simulink model "fsk_block_implementation_0"  (R2021a)
settings: Solver=VariableStepAuto  StartTime=0.0  StopTime=10  RelTol=1e-3
libraries: commchan3 x4, commsink2 x4, commdigbbndfm2 x4, commdigbbndpm3 x2, commdigbbndam3 x2, dspquant2 x2, commsrccod2 x1, dspsrcs4 x1, commrandsrc3 x1, dspsigops x1
settings Model: Creator=Yash  LastModifiedBy=Bharat Gunhalkar

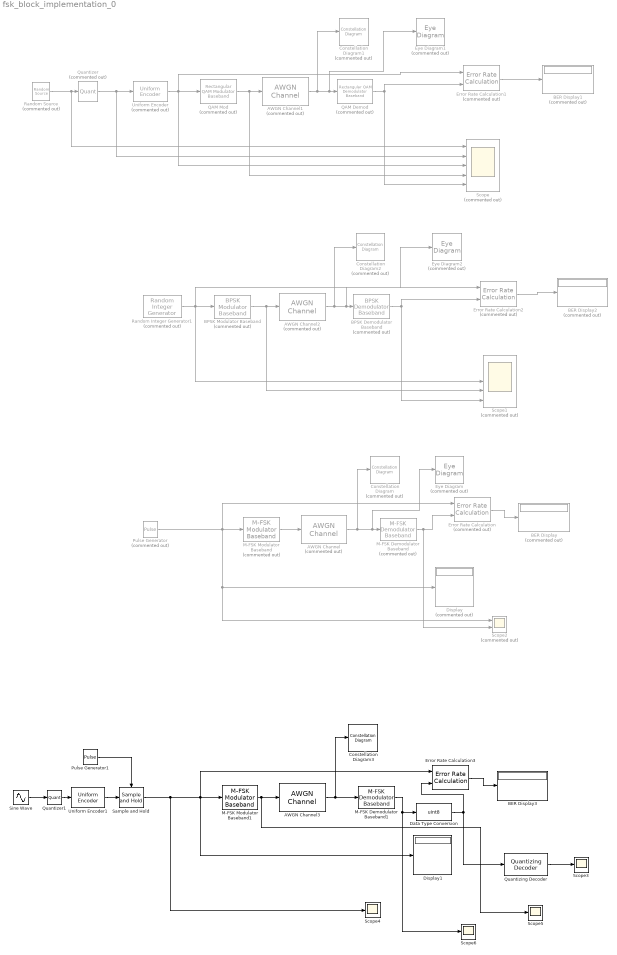
== system fsk_block_implementation_0 ==
  AWGN Channel : commchan3/AWGN Channel  Commented=on  InputProcessing=Columns as channels (frame based)  seed=67  noiseMode="Signal to noise ratio  (Eb/No)"  EbNodB=100  EsNodB=10  SNRdB=10  bitsPerSym=1  Ps=1  Tsym=1  variance=1
  AWGN Channel1 : commchan3/AWGN Channel  Commented=on  InputProcessing=Columns as channels (frame based)  seed=67  noiseMode="Signal to noise ratio  (Eb/No)"  EbNodB=-10  EsNodB=10  SNRdB=10  bitsPerSym=1  Ps=1  Tsym=1  variance=1
  AWGN Channel2 : commchan3/AWGN Channel  Commented=on  InputProcessing=Columns as channels (frame based)  seed=67  noiseMode="Signal to noise ratio  (Eb/No)"  EbNodB=-10  EsNodB=10  SNRdB=10  bitsPerSym=1  Ps=1  Tsym=1  variance=1
  AWGN Channel3 : commchan3/AWGN Channel  InputProcessing=Columns as channels (frame based)  seed=67  noiseMode="Signal to noise ratio  (Eb/No)"  EbNodB=100  EsNodB=10  SNRdB=10  bitsPerSym=1  Ps=1  Tsym=1  variance=1
  BER Display : Display  Commented=on
  BER Display1 : Display  Commented=on
  BER Display2 : Display  Commented=on
  BER Display3 : Display
  BPSK Demodulator Baseband : commdigbbndpm3/BPSK Demodulator Baseband  Commented=on  DecType=Hard decision  VarSource=Dialog  Variance=1  Ph=0  outDtype=Inherit via internal rule  derotateFactorWordLen=16  derotateFactorDataTypeStr=Inherit: Same word length as input  derotateFactorLastDataTypeStr=Inherit: Same word length as input
  BPSK Modulator Baseband : commdigbbndpm3/BPSK Modulator Baseband  Commented=on  Ph=0  outDtype=double  outWordLen=16  outUDDataType=sfix(16)  outFracLenMode=Best precision  outFracLen=15  outDataTypeStr=double  outLastDataTypeStr=double
  Constellation Diagram : ConstellationDiagram  Commented=on
  Constellation Diagram1 : ConstellationDiagram  Commented=on
  Constellation Diagram2 : ConstellationDiagram  Commented=on
  Constellation Diagram3 : ConstellationDiagram
  Data Type Conversion : DataTypeConversion  OutDataTypeStr=uint8
  Display : Display  Commented=on
  Display1 : Display
  Error Rate Calculation : commsink2/Error Rate Calculation  Commented=on  N=0  st_delay=0  cp_mode=Entire frame  subframe=[]  PMode=Port  WsName=ErrorVec  RsMode2=off  stop=off  numErr=100  maxBits=1e6
  Error Rate Calculation1 : commsink2/Error Rate Calculation  Commented=on  N=0  st_delay=0  cp_mode=Entire frame  subframe=[]  PMode=Port  WsName=ErrorVec  RsMode2=off  stop=off  numErr=100  maxBits=1e6
  Error Rate Calculation2 : commsink2/Error Rate Calculation  Commented=on  N=0  st_delay=0  cp_mode=Entire frame  subframe=[]  PMode=Port  WsName=ErrorVec  RsMode2=off  stop=off  numErr=100  maxBits=1e6
  Error Rate Calculation3 : commsink2/Error Rate Calculation  N=0  st_delay=0  cp_mode=Entire frame  subframe=[]  PMode=Port  WsName=ErrorVec  RsMode2=off  stop=off  numErr=100  maxBits=1e6
  Eye Diagram : EyeDiagram  Commented=on
  Eye Diagram1 : EyeDiagram  Commented=on
  Eye Diagram2 : EyeDiagram  Commented=on
  M-FSK Demodulator Baseband : commdigbbndfm2/M-FSK Demodulator Baseband  Commented=on  M=8  OutType=Integer  Dec=Gray  freqSep=6  numSamp=17  RateOptions=Enforce single-rate processing  outDataType=double
      settings: SourceProductBaseCode=CM
  M-FSK Demodulator Baseband1 : commdigbbndfm2/M-FSK Demodulator Baseband  M=8  OutType=Integer  Dec=Gray  freqSep=6  numSamp=17  RateOptions=Enforce single-rate processing  outDataType=double
      settings: SourceProductBaseCode=CM
  M-FSK Modulator Baseband : commdigbbndfm2/M-FSK Modulator Baseband  Commented=on  M=8  InType=Integer  Enc=Gray  freqSep=6  phaseType=Continuous  numSamp=17  RateOptions=Enforce single-rate processing  outDataType=double
  M-FSK Modulator Baseband1 : commdigbbndfm2/M-FSK Modulator Baseband  M=8  InType=Integer  Enc=Gray  freqSep=6  phaseType=Continuous  numSamp=17  RateOptions=Enforce single-rate processing  outDataType=double
  Pulse Generator : DiscretePulseGenerator  Commented=on  Amplitude=5  SampleTime=0.0001
  Pulse Generator1 : DiscretePulseGenerator  SampleTime=0.001
  QAM Demod : commdigbbndam3/Rectangular QAM Demodulator Baseband  Commented=on  M=16  OutType=Integer  DecType=Hard decision  VarSource=Dialog  Variance=1  Dec=Gray  Mapping=[0:15]  PowType=Min. distance between symbols  MinDist=2  AvgPow=1  PeakPow=1  Ph=0  outDtype1=Inherit via internal rule  outDtype2=Inherit via internal rule  derotateFactorWordLen=16  derotateFactorDataTypeStr=Inherit: Same word length as input  derotateFactorLastDataTypeStr=Inherit: Same word length as input  denormFactorWordLen=16  denormFactorDataTypeStr=Inherit: Same word length as input  denormFactorLastDataTypeStr=Inherit: Same word length as input  prodOutWordLen=32  prodOutOverflowMode=Wrap  prodOutRoundingMode=Floor  prodOutOvFlMode=off  prodOutOvFlModeLastStrValue=off  sumWordLen=32
  QAM Mod : commdigbbndam3/Rectangular QAM Modulator Baseband  Commented=on  M=16  InType=Integer  Enc=Gray  Mapping=[0:15]  PowType=Min. distance between symbols  MinDist=2  AvgPow=1  PeakPow=1  Ph=0  outDtype=double  outWordLen=16  outUDDataType=sfix(16)  outFracLenMode=Best precision  outFracLen=15  outDataTypeStr=double  outLastDataTypeStr=double
  Quantizer : Quantizer  Commented=on  QuantizationInterval=0.25  LinearizeAsGain=off
  Quantizer1 : Quantizer  QuantizationInterval=.333
  Quantizing Decoder : commsrccod2/Quantizing Decoder  codebook=[-.825 -.5 0, .5 .825]  QuDType=double
      settings: SourceProductBaseCode=CM
  Random Source : dspsrcs4/Random Source  Commented=on  SrcType=Uniform  NormMethod=Ziggurat  CltLength=12  MinVal=0  MaxVal=1  MeanVal=0  VarVal=1  RepMode=Not repeatable  rawSeed=1  IsInherit=off  SampMode=Discrete  SampTime=0.1  SampFrame=1  DataType=Single  OutComplex=Real  OutputFrames=off
  Random Integer Generator1 : commrandsrc3/Random Integer Generator  Commented=on  SetSize=2  SeedSource=Auto  Seed=0  SampleTime=0.1  SamplesPerFrame=1  OutputDataType=double  SimulateUsing=Interpreted execution
  Sample and Hold : dspsigops/Sample and Hold  trig=Rising edge  initCond=0  latchinput=off
  Scope : Scope  Commented=on  NumInputPorts=5
  Scope1 : Scope  Commented=on  NumInputPorts=5
  Scope2 : Scope  Commented=on  NumInputPorts=2
  Scope{3..6} (4 alike) : Scope
  Sine Wave : Sin  Amplitude=5  Frequency=2*pi  SampleTime=0.001
  Uniform Encoder : dspquant2/Uniform Encoder  Commented=on  peak=1  bits=4  otype=Unsigned integer
  Uniform Encoder1 : dspquant2/Uniform Encoder  peak=1  bits=3  otype=Unsigned integer
  wires:
  Error Rate Calculation1/1 -> BER Display1/1
  QAM Mod/1 -> AWGN Channel1/1, Scope/4
  Quantizer/1 -> Uniform Encoder/1, Scope/2
  AWGN Channel1/1 -> Eye Diagram1/1, QAM Demod/1, Constellation Diagram1/1
  Uniform Encoder/1 -> QAM Mod/1, Error Rate Calculation1/1, Scope/3
  Random Source/1 -> Scope/1, Quantizer/1
  QAM Demod/1 -> Error Rate Calculation1/2, Scope/5
  Random Integer Generator1/1 -> BPSK Modulator Baseband/1, Error Rate Calculation2/1, Scope1/3
  AWGN Channel2/1 -> BPSK Demodulator Baseband/1, Eye Diagram2/1, Constellation Diagram2/1
  Error Rate Calculation2/1 -> BER Display2/1
  BPSK Demodulator Baseband/1 -> Error Rate Calculation2/2, Scope1/5
  BPSK Modulator Baseband/1 -> AWGN Channel2/1, Scope1/4
  AWGN Channel/1 -> Eye Diagram/1, M-FSK Demodulator Baseband/1, Constellation Diagram/1
  M-FSK Demodulator Baseband/1 -> Scope2/2, Error Rate Calculation/2
  Error Rate Calculation/1 -> BER Display/1
  Pulse Generator/1 -> Scope2/1, Display/1, Error Rate Calculation/1, M-FSK Modulator Baseband/1
  M-FSK Modulator Baseband/1 -> AWGN Channel/1
  Sample and Hold/1 -> Scope4/1, Display1/1, Error Rate Calculation3/1, M-FSK Modulator Baseband1/1
  Error Rate Calculation3/1 -> BER Display3/1
  AWGN Channel3/1 -> M-FSK Demodulator Baseband1/1, Constellation Diagram3/1
  M-FSK Demodulator Baseband1/1 -> Scope6/1, Data Type Conversion/1
  M-FSK Modulator Baseband1/1 -> Scope5/1, AWGN Channel3/1
  Sine Wave/1 -> Quantizer1/1
  Quantizer1/1 -> Uniform Encoder1/1
  Uniform Encoder1/1 -> Sample and Hold/1
  Pulse Generator1/1 -> Sample and Hold/Trigger
  Data Type Conversion/1 -> Quantizing Decoder/1, Error Rate Calculation3/2
  Quantizing Decoder/1 -> Scope3/1
